simulink model "Gainsimulink"  (R2017a)
settings: Solver=VariableStepAuto  StartTime=0.0  StopTime=10.0  RelTol=1e-3
settings Model: Creator=Administrator  LastModifiedBy=Administrator

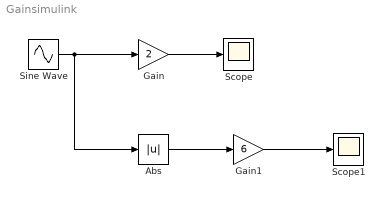
== system Gainsimulink ==
  Abs : Abs
  Gain : Gain  Gain=2
  Gain1 : Gain  Gain=6
  Scope : Scope
  Scope1 : Scope
  Sine Wave : Sin  SampleTime=0
  wires:
  Sine Wave/1 -> Abs/1, Gain/1
  Gain/1 -> Scope/1
  Abs/1 -> Gain1/1
  Gain1/1 -> Scope1/1
